simulink model "legstatespacemodel"  (R2022b)
settings: Solver=VariableStepAuto  StartTime=0.0  StopTime=1.5  FixedStep=1e-6  RelTol=1e-3
values from neighbouring files (symbols this model uses):
  A = params.state_space.state_matrix    [Kalman_sim.m]    (also in param2.m = [ 0   1    0; parameter.m = [ 0   1    0   0)
  B = params.state_space.input_matrix    [Kalman_sim.m]    (also in param2.m = [0; parameter.m = [0)
  b = Vmax*a    (= 3.6)    [ElbowKNES300.m]    (also in Kalman_sim.m = 0.00140884756269; elbow.m = pars(19); parameter.m = 0.01)
  C = params.state_space.output_matrix    [Kalman_sim.m]    (also in param2.m = [1 0 0]; parameter.m = [0  0  1  0])
  D = params.state_space.feedthrough_matrix    [Kalman_sim.m]    (also in param2.m = [0]; parameter.m = [0])
  Ip = Ips + Mp * L^2    (= 0.06775)    [parameter.m]
libraries: dspsrcs4 x1, slpidlib x1
settings Model: Creator=Electrical  LastModifiedBy=User
settings SolverCC: AlgebraicLoopSolver=TrustRegion
settings DataIOCC: ReturnWorkspaceOutputs=off
settings DebuggingCC: UnconnectedInputMsg=warning  UnconnectedOutputMsg=warning  UnconnectedLineMsg=warning  SFMachineParentedDataDiag=warning  ArithmeticOperatorsInVariantConditions=warning
settings ModelReferenceCC: EnableRefExpFcnMdlSchedulingChecks=on
settings SFSimCC: SimUseLocalCustomCode=off  CustomCodeUndefinedFunction=UseInterfaceOnly
settings RTWCC: RTWUseLocalCustomCode=off

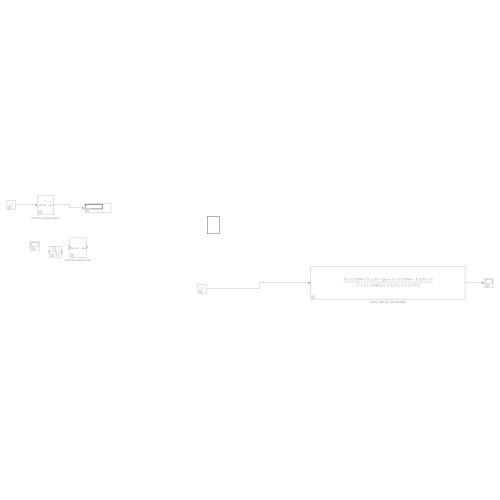
[thumbnail: Simulink's stored preview of the top-level diagram]
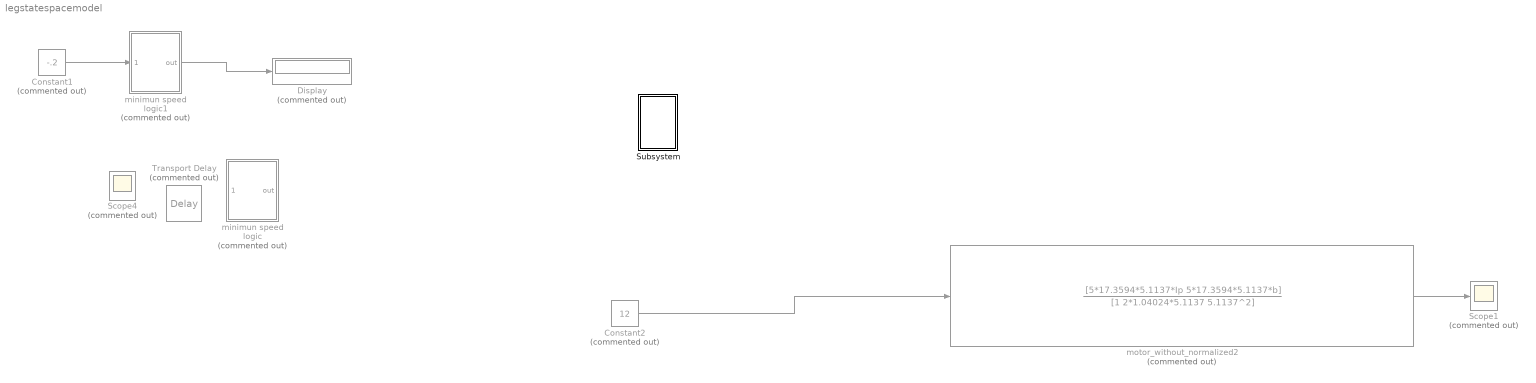
== system legstatespacemodel ==
  Constant1 : Constant  Commented=on  Value=-.2
  Constant2 : Constant  Commented=on  Value=12
  Display : Display  Commented=on
  Scope1 : Scope  Commented=on
  Scope4 : Scope  Commented=on
  Subsystem : Subsystem
  Transport Delay : TransportDelay  Commented=on  DelayTime=0.1
  minimun speed logic : Subsystem  Commented=on
  minimun speed logic1 : Subsystem  Commented=on
  motor_without_normalized2 : TransferFcn  Commented=on  Numerator=[5*17.3594*5.1137*Ip 5*17.3594*5.1137*b]  Denominator=[1 2*1.04024*5.1137 5.1137^2]
  wires:
  Constant1/1 -> minimun speed logic1/1(pid val)
  minimun speed logic1/1(out) -> Display/1
  Constant2/1 -> motor_without_normalized2/1
  motor_without_normalized2/1 -> Scope1/1

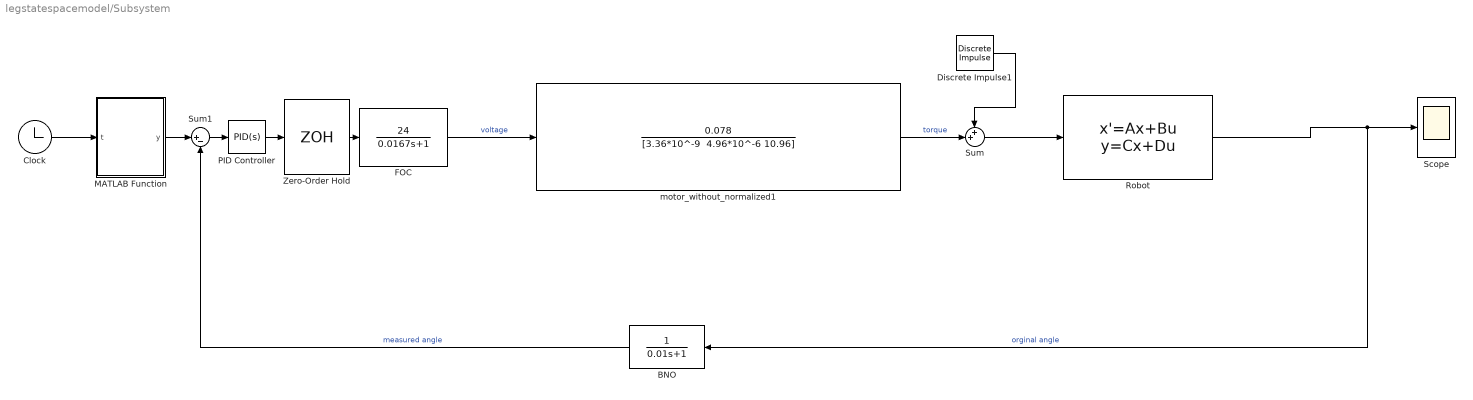
== system legstatespacemodel/Subsystem ==
  BNO : TransferFcn  Denominator=[0.01 1]
  Clock : Clock
  Discrete Impulse1 : dspsrcs4/Discrete  Impulse  Delay=0  SampleTime=1  FrameSample=1  OutputFrames=off  dataType=double  isSigned=on  wordLen=16  udDataType=sfix(16)  fracBitsMode=Best precision  numFracBits=15  OutDataTypeStr=double  LastOutDataTypeStr=double
  FOC : TransferFcn  Numerator=[24]  Denominator=[0.0167 1]
  MATLAB Function : MATLAB Function  TreatAsAtomicUnit=on
  PID Controller : slpidlib/PID Controller  Controller=PID  Form=Parallel  TimeDomain=Continuous-time  UseExternalTs=off  SampleTime=-1  IntegratorMethod=Trapezoidal  FilterMethod=Backward Euler  ControllerParametersSource=internal  P=10  I=30  UseKiTs=off  D=15  N=100  UseFilter=on  TunerSelectOption=Transfer Function Based (PID Tuner App)  InitialConditionSource=internal  InitialConditionForIntegrator=0  InitialConditionForFilter=0  DifferentiatorICPrevScaledInput=0  ExternalReset=none  TrackingMode=off  Kt=1  LimitOutput=off  SatLimitsSource=internal  UpperSaturationLimit=1  LowerSaturationLimit=-1  LinearizeAsGain=off  AntiWindupMode=back-calculation  Kb=0.01  LimitIntegrator=off  UpperIntegratorSaturationLimit=inf  LowerIntegratorSaturationLimit=-inf  POutMin=[]  POutMax=[]  IOutMin=[]  IOutMax=[]  DOutMin=[]  DOutMax=[]  NOutMin=[]  NOutMax=[]  SumOutMin=[]  SumOutMax=[]  SaturationOutMin=[]  SaturationOutMax=[]  PParamMin=[]  PParamMax=[]  IParamMin=[]  IParamMax=[]  DParamMin=[]  DParamMax=[]  NParamMin=[]  NParamMax=[]  KbParamMin=[]  KbParamMax=[]  KtParamMin=[]  KtParamMax=[]  KbOutMin=[]  KbOutMax=[]  KtOutMin=[]  KtOutMax=[]  IntegratorOutMin=[]  IntegratorOutMax=[]  FilterOutMin=[]  FilterOutMax=[]  SumI1OutMin=[]  SumI1OutMax=[]  SumI2OutMin=[]  SumI2OutMax=[]  SumI3OutMin=[]  SumI3OutMax=[]  SumI4OutMin=[]  SumI4OutMax=[]  SumDOutMin=[]  SumDOutMax=[]  DifferentiatorOutMin=[]  DifferentiatorOutMax=[]  FilterDiffOutCoefMin=[]  FilterDiffOutCoefMax=[]  ReciprocalOutMin=[]  ReciprocalOutMax=[]  SumDenOutMin=[]  SumDenOutMax=[]  SumNumOutMin=[]  SumNumOutMax=[]  DivideOutMin=[]  DivideOutMax=[]  UdiffTsProdOutMin=[]  UdiffTsProdOutMax=[]  NTsProdOutMin=[]  NTsProdOutMax=[]  UintegralTsProdOutMin=[]  UintegralTsProdOutMax=[]  UngainTsProdOutMin=[]  UngainTsProdOutMax=[]  ClampingZeroOutDataTypeStr=Inherit: Inherit via back propagation  ClampingZeroOutMin=[]  ClampingZeroOutMax=[]  FilterDenConstantOutDataTypeStr=Inherit: Inherit via back propagation  FilterDenConstantOutMin=[]  FilterDenConstantOutMax=[]  PCopyOutDataTypeStr=Inherit: Inherit via back propagation  PCopyOutMin=[]  PCopyOutMax=[]  NCopyOutDataTypeStr=Inherit: Inherit via back propagation  NCopyOutMin=[]  NCopyOutMax=[]  IntegratorContinuousStateAttributes=''  IntegratorStateMustResolveToSignalObject=off  IntegratorRTWStateStorageClass=Auto  FilterContinuousStateAttributes=''  FilterStateMustResolveToSignalObject=off  FilterRTWStateStorageClass=Auto  ParallelPVariant=InternalParameters  IdealPVariant=Disabled  IVariant=InternalParameters  DVariant=InternalParameters  IntegratorVariant=Continuous  SatVariant=Disabled  AWVariant=Passthrough  PCopyVariant=Disabled  TRVariant=Disabled  FdbkBlocksVariant=Forward  IdealPFdbkVariant=Disabled  SatFdbkVariant=Disabled  DerivativeFilterVariant=ContFilter  NVariant=InternalParameters  NCopyVariant=Disabled  FilterICVariant=InternalICsFilter  IntegratorICVariant=InternalICs  ExternalResetVariant=Disabled  TRSumVariant=Passthrough  SumFdbkVariant=Disabled  SumVariant=Sum_PID  TsampFilterVariant=InternalTs  TsampNgainVariant=Passthrough  TsampIntegralVariant=Passthrough  ExternalSaturationOutDataTypeStr=Inherit: Same as second input
  Robot : StateSpace  A=A  B=B  C=C  D=D  InitialCondition=0
  Scope : Scope
  Sum : Sum  Inputs=++|
  Sum1 : Sum  Inputs=|+-
  Zero-Order Hold : ZeroOrderHold  SampleTime=30/1000
  motor_without_normalized1 : TransferFcn  Numerator=[0.078]  Denominator="[3.36*10^-9  4.96*10^-6 10.96]"
  wires:
  Sum/1 -> Robot/1
  motor_without_normalized1/1 -> Sum/2  "torque"
  FOC/1 -> motor_without_normalized1/1  "voltage"
  Zero-Order Hold/1 -> FOC/1
  Clock/1 -> MATLAB Function/1(t)
  Discrete Impulse1/1 -> Sum/1
  PID Controller/1 -> Zero-Order Hold/1
  BNO/1 -> Sum1/2  "measured angle"
  MATLAB Function/1(y) -> Sum1/1
  Sum1/1 -> PID Controller/1
  Robot/1 -> BNO/1, Scope/1  "orginal angle"

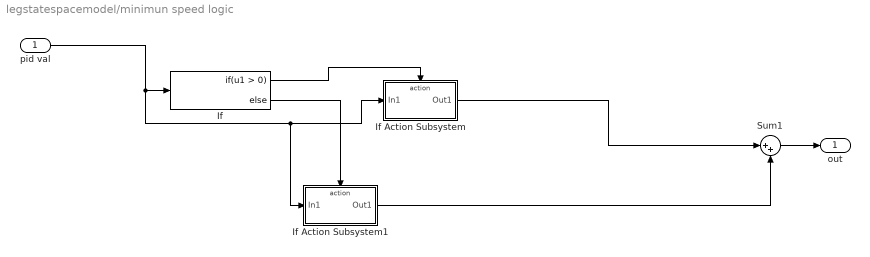
== system legstatespacemodel/minimun speed logic ==
  pid val : Inport
  If : If
  If Action Subsystem : Subsystem  TreatAsAtomicUnit=on
  If Action Subsystem1 : Subsystem  TreatAsAtomicUnit=on
  Sum1 : Sum  Inputs=|++
  out : Outport  VectorParamsAs1DForOutWhenUnconnected=off
  wires:
  pid val/1 -> If/1, If Action Subsystem1/1(In1), If Action Subsystem/1(In1)
  If/1 -> If Action Subsystem/Action
  Sum1/1 -> out/1
  If/2 -> If Action Subsystem1/Action
  If Action Subsystem1/1(Out1) -> Sum1/2
  If Action Subsystem/1(Out1) -> Sum1/1

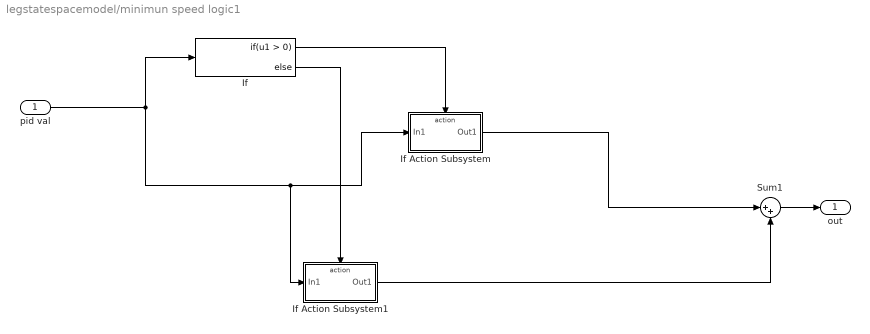
== system legstatespacemodel/minimun speed logic1 ==
  pid val : Inport
  If : If
  If Action Subsystem : Subsystem  TreatAsAtomicUnit=on
  If Action Subsystem1 : Subsystem  TreatAsAtomicUnit=on
  Sum1 : Sum  Inputs=|++
  out : Outport  VectorParamsAs1DForOutWhenUnconnected=off
  wires:
  If Action Subsystem/1(Out1) -> Sum1/1
  If Action Subsystem1/1(Out1) -> Sum1/2
  If/2 -> If Action Subsystem1/Action
  Sum1/1 -> out/1
  If/1 -> If Action Subsystem/Action
  pid val/1 -> If Action Subsystem/1(In1), If Action Subsystem1/1(In1), If/1

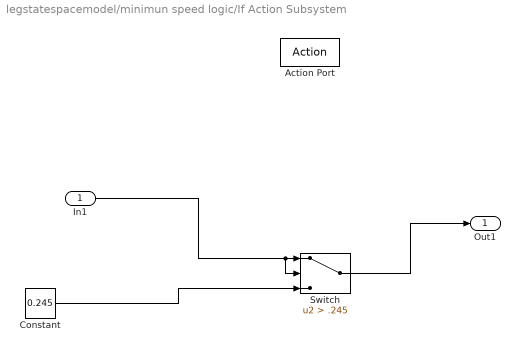
== system legstatespacemodel/minimun speed logic/If Action Subsystem ==
  In1 : Inport
  Action Port : ActionPort
  Constant : Constant  Value=0.245
  Switch : Switch  Criteria=u2 > Threshold  Threshold=.245  SaturateOnIntegerOverflow=off  InputSameDT=off
  Out1 : Outport  VectorParamsAs1DForOutWhenUnconnected=off
  wires:
  Switch/1 -> Out1/1
  Constant/1 -> Switch/3
  In1/1 -> Switch/2, Switch/1

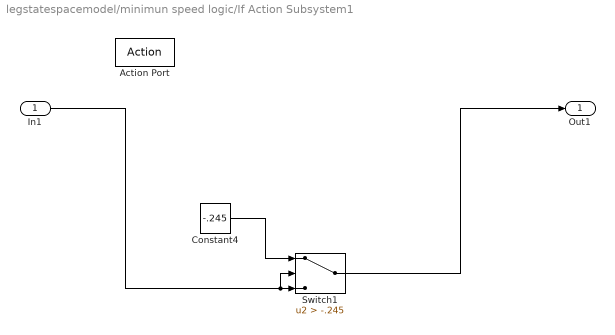
== system legstatespacemodel/minimun speed logic/If Action Subsystem1 ==
  In1 : Inport
  Action Port : ActionPort
  Constant4 : Constant  Value=-.245
  Switch1 : Switch  Criteria=u2 > Threshold  Threshold=-.245  SaturateOnIntegerOverflow=off  InputSameDT=off
  Out1 : Outport  VectorParamsAs1DForOutWhenUnconnected=off
  wires:
  In1/1 -> Switch1/2, Switch1/3
  Constant4/1 -> Switch1/1
  Switch1/1 -> Out1/1

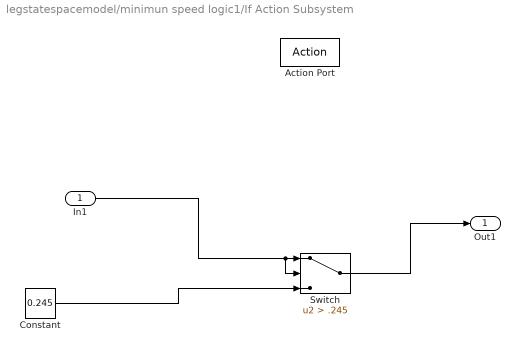
== system legstatespacemodel/minimun speed logic1/If Action Subsystem ==
  In1 : Inport
  Action Port : ActionPort  ActionPortLabel=if { }
  Constant : Constant  Value=0.245
  Switch : Switch  Criteria=u2 > Threshold  Threshold=.245  SaturateOnIntegerOverflow=off  InputSameDT=off
  Out1 : Outport  VectorParamsAs1DForOutWhenUnconnected=off
  wires:
  In1/1 -> Switch/1, Switch/2
  Constant/1 -> Switch/3
  Switch/1 -> Out1/1

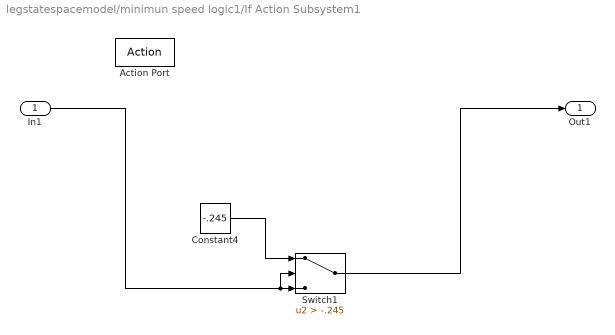
== system legstatespacemodel/minimun speed logic1/If Action Subsystem1 ==
  In1 : Inport
  Action Port : ActionPort  ActionPortLabel=else { }
  Constant4 : Constant  Value=-.245
  Switch1 : Switch  Criteria=u2 > Threshold  Threshold=-.245  SaturateOnIntegerOverflow=off  InputSameDT=off
  Out1 : Outport  VectorParamsAs1DForOutWhenUnconnected=off
  wires:
  Switch1/1 -> Out1/1
  Constant4/1 -> Switch1/1
  In1/1 -> Switch1/3, Switch1/2

== matlab function legstatespacemodel/Subsystem/MATLAB Function ==
  data: t input; y output
function y = fourier_signal(t)
    % Load data from file
    f_k = load('data.txt');
    
    % Define parameters
    M = length(f_k);
    stride_points = 150;
    sampling_freq = 100;  
    delta_t = 1 / sampling_freq;
    T = stride_points * delta_t;  
    N = 7; % Number of harmonics

    % Fourier Coefficients Calculation
    a0 = mean(f_k);
    a_n = zeros(1, N);
    b_n = zeros(1, N);
    omega_n = 2 * pi / T;
    
    for n = 1:N
        a_n(n) = (2 / M) * sum(f_k .* cos(omega_n * n * (0:M-1)' * delta_t));
        b_n(n) = (2 / M) * sum(f_k .* sin(omega_n * n * (0:M-1)' * delta_t));
    end

    % Reconstruct the signal
    y = a0 / 2; % DC component
    for n = 1:N
        y = y + a_n(n) * cos(omega_n * n * t) + b_n(n) * sin(omega_n * n * t);
    end
end
